simulink library "Acceleration_Calculation"  (R2019b)
settings: Solver=VariableStepAuto  StartTime=0.0  StopTime=10.0  RelTol=1e-3
undefined symbols (not defined in the file): DiscIntNeverNeededParam
settings Model: Creator=Alexander Koch  LastModifiedBy=ga69qig
settings DataIOCC: ReturnWorkspaceOutputs=off
settings DebuggingCC: ArithmeticOperatorsInVariantConditions=warning
settings SFSimCC: SimUseLocalCustomCode=off  CustomCodeUndefinedFunction=UseInterfaceOnly
settings RTWCC: RTWUseLocalCustomCode=off
settings CodeAppCC: StateflowObjectComments=on

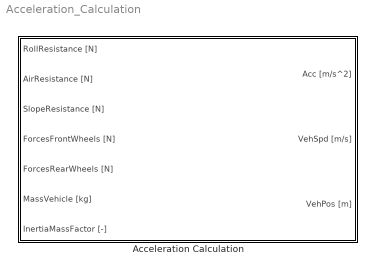
== system Acceleration_Calculation ==
  Acceleration Calculation : Subsystem  mask(SB){InitialCondition=0, LocalSampleTime=-1}
      mask prompts: InitialCondition "Initial Speed [m/s]"; LocalSampleTime "Local System Sample-Time [s]"
      mask help:
      | <Author> Alexander Koch, Benedikt Danquah based on Stefan Müller [1], Stephan Rohr [2]  </Author>
      | <Date> 21/03/2017 </Date>
      | <Sources>
      | [1] S. Mueller, S. Rohr, und et al, Hrsg, Analysing the Influence of Driver Behaviour and Tuning Measures on Battery Aging and Residual Value of Electric Vehicles, 2017
      | </Sources>
      |
      | <Description>
      | Requires roll resistance, air resistance, slope resistance, forces at front and rear wheels and the mass of the vehicle. Through an inertia mass factor which represents the throwing body, an acceleration is calculated. Through integration, the vehicle speed and position is calculated. negative speeds are filtered out.
      | </Description>
      mask init:
      | GlobalSampleTime = CalcGlobalSampleTime(LocalSampleTime);
      mask Help:
      | <Parameters>
      | Inertia Mass Factor [-]
      | 	<Min> 1 </Min>
      | Local System Sample-Time [s]
      | 	<Min> GlobalSampleTime </Min>
      | Global Sample-Time [s]
      | </Parameters>
      | 
      | <Inputs>
      | RollResistance [N]
      | 	<sign orientation> [+] slows down </sign orientation>
      | AirResistance [N]
      | 	<sign orientation> [+] slows down </sign orientation>
      | SlopeResistance [N]
      | 	<sign orientation> [+] slows down </sign orientation>
      | ForcesFrontWheels [N]
      | 	<sign orientation> [+] accelerates </sign orientation>
      | ForcesRearWheels [N]
      | 	<sign orientation> [+] accelerates </sign orientation>
      | </Inputs>
      | 
      | <Outputs>
      | Acc [m/s^2]
      | VehSpd [m/s]
      | 	<Min> 0 </Min>
      | VehPos [m]
      | 	<Min> 0 </Min>
      | </Outputs>
      | <Sources>
      | [1] S. Mueller, S. Rohr, W. Schmid, and M. Lienkamp, “Analysing the Influence of Driver Behaviour and Tuning Measures on Battery Aging and Residual Value of Electric Vehicles,” in Proc. EVS30 Symposium, Stuttgart, 2017, pp. 1–12.
      | [2] S. Rohr, “Technisch-wirtschaftliche Analyse des Zweitnutzungs- potentials von Lithium-Ionen-Traktionsbatterien,” Dissertation, Institute of Automotive Technology, Technical University Munich, Munich, 2018.
      | </Sources>
      mask TypeOptions InitialCondition:
      | Discrete-Time
      | Integrator/InitialCondition
      mask TypeOptions LocalSampleTime: RollResistance [N]/SampleTime | AirResistance [N]/SampleTime | SlopeResistance [N]/SampleTime | ForcesFrontWheels [N]/SampleTime | ForcesRearWheels [N]/SampleTime | MassVehicle [kg]/SampleTime | InertiaMassFactor [-]/SampleTime
      mask DialogControl Container4 Prompt: Documentation:
      mask DialogControl Control2 Prompt: %<MaskHelp>
      mask DialogControl Container3 Prompt: Parameter
      mask DialogControl Container5 Prompt: Sample Time
      mask Display:
      | [picturexpos,pictureypos,picturewidth,pictureheight] = ...
      |     CalcBlockPicturePosition(gcb,1,0.01,0.1,100,80); % calculating picture position depending on Block size and minimum margin size
      | image('Acceleration_Calculation.svg',[picturexpos pictureypos picturewidth pictureheight]); % plot picture to block

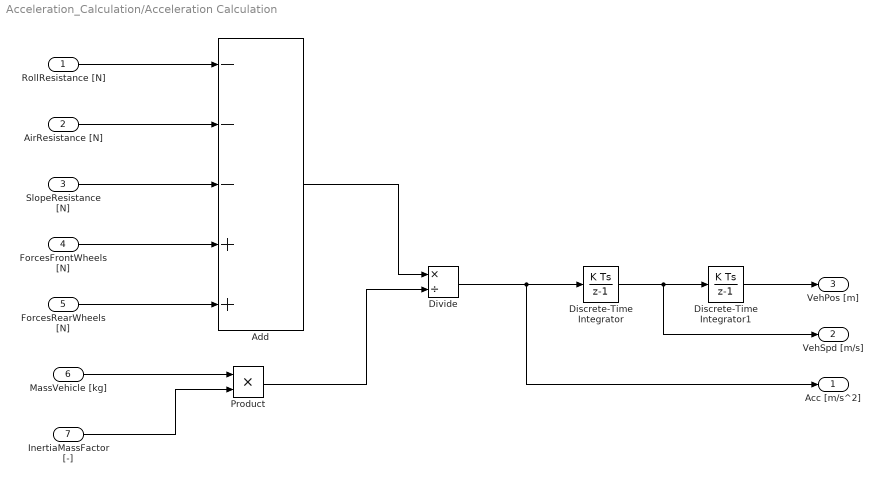
== system Acceleration_Calculation/Acceleration Calculation ==
  RollResistance [N] : Inport  SampleTime=LocalSampleTime
  AirResistance [N] : Inport  Port=2  SampleTime=LocalSampleTime
  SlopeResistance [N] : Inport  Port=3  SampleTime=LocalSampleTime
  ForcesFrontWheels [N] : Inport  Port=4  SampleTime=LocalSampleTime
  ForcesRearWheels [N] : Inport  Port=5  SampleTime=LocalSampleTime
  MassVehicle [kg] : Inport  Port=6  SampleTime=LocalSampleTime
  InertiaMassFactor [-] : Inport  Port=7  SampleTime=LocalSampleTime
  Add : Sum  Inputs=---++
  Discrete-Time Integrator : DiscreteIntegrator  InitialCondition=InitialCondition  SampleTime=-1  LimitOutput=on  LowerSaturationLimit=0  ICPrevOutput=DiscIntNeverNeededParam  ICPrevScaledInput=DiscIntNeverNeededParam
  Discrete-Time Integrator1 : DiscreteIntegrator  SampleTime=-1  ICPrevOutput=DiscIntNeverNeededParam  ICPrevScaledInput=DiscIntNeverNeededParam
  Divide : Product  Inputs=*/
  Product : Product
  Acc [m/s^2] : Outport  SampleTime=GlobalSampleTime  VectorParamsAs1DForOutWhenUnconnected=off
  VehSpd [m/s] : Outport  Port=2  SampleTime=GlobalSampleTime  VectorParamsAs1DForOutWhenUnconnected=off
  VehPos [m] : Outport  Port=3  SampleTime=GlobalSampleTime  VectorParamsAs1DForOutWhenUnconnected=off
  wires:
  AirResistance [N]/1 -> Add/2
  MassVehicle [kg]/1 -> Product/1
  RollResistance [N]/1 -> Add/1
  SlopeResistance [N]/1 -> Add/3
  ForcesFrontWheels [N]/1 -> Add/4
  ForcesRearWheels [N]/1 -> Add/5
  Discrete-Time Integrator1/1 -> VehPos [m]/1
  Discrete-Time Integrator/1 -> VehSpd [m/s]/1, Discrete-Time Integrator1/1
  Divide/1 -> Acc [m/s^2]/1, Discrete-Time Integrator/1
  Product/1 -> Divide/2
  Add/1 -> Divide/1
  InertiaMassFactor [-]/1 -> Product/2
